simulink model "AOTRT"  (R2017b)
settings: Solver=FixedStepDiscrete  StartTime=0  StopTime=5  FixedStep=0.001  MaxStep=0.001  RelTol=1e-3  EnableMultiTasking=on
model workspace (MAT data in the model file):
  Occurrence.FaultRemote = 1
  Occurrence.FaultLow = 2
  Occurrence.FaultLow_2 = 3
  Occurrence.FaultModerate = 4
  Occurrence.FaultModerate_2 = 5
  Occurrence.FaultModerate_3 = 6
  Occurrence.FaultHigh = 7
  Occurrence.FaultHigh_2 = 8
  Occurrence.Tolerance = 9
  Occurrence.OK = 10
  Partitions.Last = ''
  Partitions.All = '*'
  Severity.OK = 0
  Severity.Warn = 1
  Severity.VeryMinor = 2
  Severity.Minor = 3
  Severity.VeryLow = 4
  Severity.Low = 5
  Severity.Moderate = 6
  Severity.High = 7
  Severity.VeryHigh = 8
  Severity.HazardousWithWarning = 9
  Severity.HazardousNoWarning = 10
  Severity.Error = 11
  Severity.ErrorFatal = 20
  block : handle (value not decoded)
  t = 0
  time = 0
libraries: EPS_lib x1
settings Model: RequirementInfo={'linktype_rmi_url' 'easee:VCC_EEDM,8630600' '' 'true' 'REQPROD 431295 / MAIN ; 5 : Actions on Torque Request timeout' '' } %GIDa_82bd7b7d_6f03_44d5_8654_a9f9591c358b  conn_id=-1  report_delay=1  Creator=aande176  LastModifiedBy=JEDDELAN
settings SolverCC: AutoInsertRateTranBlk=on
settings DataIOCC: ExternalInput=[],CPSRSts__CPSRSts,[],[],[],[],[],[],[],LvTestSts__LvTestSts,IsgPwrLimMin__IsgPwrLimMin,[],IsgPwrLimMax__IsgPwrLimMax,TqAvlIntFromIfCpt__TqAvlIntFromIfCpt,[],[],[],[],[],TqAllwdInt__TqAllwdInt,[],[],[],[],[],[],[],HvBattUDynMaxLim__HvBattUDynMaxLim,[],HvBattUDynMinLim__HvBattUDynMinLim,[],InitCmpl__InitCmpl,[],[],[],[],[],[],[],[],[],[],[],HvTestSts__HvTestSts,[],[],[],IsgModReq__IsgModReq,[],[],[],[],[],[],[],[],[],[],[],[],[],[],[],[],[],EngSt1WdSts__EngSt1WdSts__IsUpdated,IsgSpdReq__IsgSpdReq__IsUpdated,IsgModReq__IsgModReq__IsUpdated,HvSysRlySts__HvSysRlySts__IsUpdated,HvSysRlySts_toController,[],[],[],[],ImobPrpsnAllwd__ImobPrpsnAllwd__dummy,[],[],[],[],ImobTurnOffAllwd__ImobTurnOffAllwd__dummy,[],[],[],No_GearEven,B_CloseClutchOdd,B_CloseClutchEven,[],[],[],B_EnableVSpAct,V_Vehicle_SetPoint_mps,[]  SaveFormat=StructureWithTime  SaveOutput=off  SignalLogging=off  DSMLogging=off  SaveTime=off  SignalLoggingName=slunit_logdata
settings OptimizationCC: DefaultParameterBehavior=Inlined  ExpressionDepthLimit=2147483647  LifeSpan=Inf
settings DebuggingCC: RTPrefix=warning  AlgebraicLoopMsg=error  CheckSSInitialOutputMsg=off  SolverPrmCheckMsg=warning  IntegerOverflowMsg=none  ParameterPrecisionLossMsg=none  FcnCallInpInsideContextMsg=warning  BusObjectLabelMismatch=error  ModelReferenceDataLoggingMessage=none  StateNameClashWarn=warning  SFUnexpectedBacktrackingDiag=warning  SFNoUnconditionalDefaultTransitionDiag=warning  SFExecutionAtInitializationDiag=none  IntegerSaturationMsg=none
settings HardwareCC: ProdBitPerLong=64  ProdHWDeviceType=Intel->x86-64
settings ModelReferenceCC: UpdateModelReferenceTargets=AssumeUpToDate  PropagateSignalLabelsOutOfModel=off
settings SFSimCC: SimGenImportedTypeDefs=on
settings RTWCC: RTWUseSimCustomCode=on
settings CodeAppCC: StateflowObjectComments=on
settings GRTTargetCC: TargetLangStandard=C89/C90 (ANSI)  GeneratePreprocessorConditionals=Disable all  CombineOutputUpdateFcns=off  GRTInterface=on
settings ConfigComp: CovScope=Subsystem  CovPath=RequirementsEvaluation/AvailableTorque  CovMetricSettings=dcw  CovHTMLOptions=-sRT=1 -aTS=1 -bRG=1 -bTC=1 -hTR=0 -nFC=0 -scm=1 -bcm=1 -xEv=0  CovHtmlReporting=on  CovSaveCumulativeToWorkspaceVar=on  CovSaveSingleToWorkspaceVar=on  CovExternalEMLEnable=off

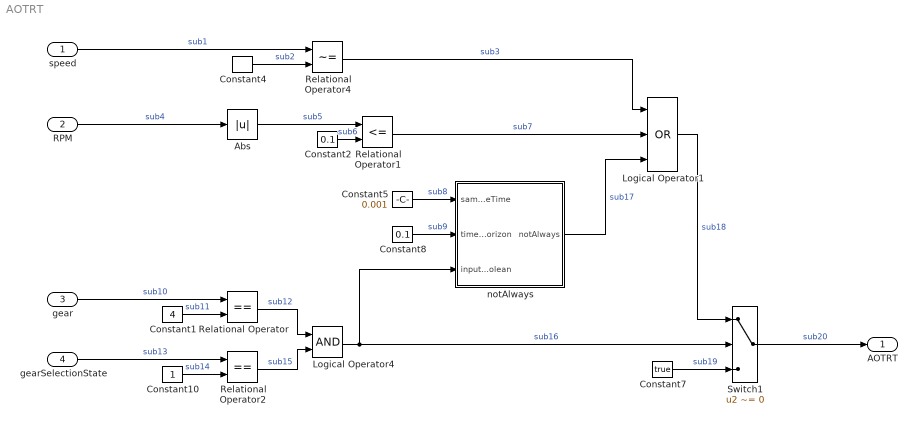
== system AOTRT ==
  speed : Inport  OutDataTypeStr=TqInt  PortDimensions=1  SampleTime=[0.001,0]
  RPM : Inport  Port=2  OutDataTypeStr=TqInt  PortDimensions=1  SampleTime=[0.001,0]
  gear : Inport  Port=3  OutDataTypeStr=Enum: ComTiOut  PortDimensions=1  SampleTime=[0.001,0]  Interpolate=off
  gearSelectionState : Inport  Port=4  OutDataTypeStr=Enum: ModSts  PortDimensions=1  SampleTime=[0.001,0]  Interpolate=off
  Abs : Abs
  Constant1 : Constant  Value=4  OutDataTypeStr=double  mask(EPS_param){param=4, displayname=4: 4}
      mask prompts: param "Parameter"; displayname "Display"
      mask help:
      | Block is used for EPS parameters.
      | Block shows the annotation 'displayname' (which is a hidden feature in the mask)
      | which is a part of the Parameter Name (if the parameter name syntax is 'ModelNameParam')
      mask init:
      | try
      |     set_param(gcb,'LinkStatus','none');
      | catch
      |     warning('Not possible to break links');
      | end
      | icondisp = 'P';
      | mdlname = regexp(get_param(gcs,'Parent'),'\w*(?=\_)','match','once');
      | name = get_param(gcb,'param');
      | 
      | objclass = evalin('base',['class(',name,')']);
      | objtype = typeobj(objclass);
      | if objtype.isenum
      |     nametype = regexp(name,'\.','split');
      | % if length(nametype) > 1
      |     % is enum
      |     displayname = nametype{2};
      |     icondisp = 'E';
      |     set_param(gcb,'OutDataTypeStr',['Enum: ',nametype{1}]);    
      | elseif isa(evalin('base',name),'AUTOSAR.Parameter')
      |     % Autosar parameter
      |     displayname = regexprep(name,mdlname,'');
      |     icondisp = 'P';
      |     set_param(gcb,'OutDataTypeStr',['Inherit: Inherit from ''Constant value''']);
      | else
      |     % regular constant
      |     displayname = [name,': ',num2str(evalin('base',name))];
      |     icondisp = 'C';
      |     if strcmp(objtype.name,'logical')
      |         set_param(gcb,'OutDataTypeStr','boolean');
      |     else
      |         set_param(gcb,'OutDataTypeStr',objtype.name);
      |     end  
      | end
      | set_param(gcb,'displayname',displayname);
      | set_param(gcb,'Value',name);
      settings: AttributesFormatString=%<displayname>
      mask Display: disp(icondisp)
  Constant10 : Constant  OutDataTypeStr=double  mask(EPS_param_v0.1){param=1, displayname=1: 1}
      mask prompts: param "Parameter"; displayname "Display"
      mask help:
      | Block is used for EPS parameters.
      | Block shows the annotation 'displayname' (which is a hidden feature in the mask)
      | which is a part of the Parameter Name (if the parameter name syntax is 'ModelNameParam')
      mask init:
      | try
      |     set_param(gcb,'LinkStatus','none');
      | catch
      |     warning('Not possible to break links');
      | end
      | icondisp = 'P';
      | mdlname = regexp(get_param(gcs,'Parent'),'\w*(?=\_)','match','once');
      | name = get_param(gcb,'param');
      | 
      | objclass = evalin('base',['class(',name,')']);
      | [enumdummy,enumList] = evalin('base',['enumeration(',name,')']);
      | if ~isempty(enumList)
      |     nametype = regexp(name,'\.','split');
      | % if length(nametype) > 1
      |     % is enum
      |     displayname = nametype{2};
      |     icondisp = 'E';
      |     set_param(gcb,'OutDataTypeStr',['Enum: ',nametype{1}]);    
      | elseif isa(evalin('base',name),'AUTOSAR.Parameter')
      |     % Autosar parameter
      |     displayname = regexprep(name,mdlname,'');
      |     icondisp = 'P';
      |     set_param(gcb,'OutDataTypeStr',['Inherit: Inherit from ''Constant value''']);
      | else
      |     % regular constant
      |     displayname = [regexprep(name,mdlname,''),': ',num2str(evalin('base',name))];
      |     icondisp = 'C';
      |     if strcmp(objclass,'logical')
      |         set_param(gcb,'OutDataTypeStr','boolean');
      |     else
      |         set_param(gcb,'OutDataTypeStr',objclass);
      |     end  
      | end
      | set_param(gcb,'displayname',displayname);
      | set_param(gcb,'Value',name);
      settings: AttributesFormatString=%<displayname>
      mask Display: disp(icondisp)
  Constant2 : Constant  Value=0.1  OutDataTypeStr=double  mask(EPS_param_v0.1){param=0.1, displayname=0.1: 0.1}
      mask prompts: param "Parameter"; displayname "Display"
      mask help:
      | Block is used for EPS parameters.
      | Block shows the annotation 'displayname' (which is a hidden feature in the mask)
      | which is a part of the Parameter Name (if the parameter name syntax is 'ModelNameParam')
      mask init: same as AOTRT/Constant10
      settings: AttributesFormatString=%<displayname>
      mask Display: disp(icondisp)
  Constant4 : EPS_lib/CalibrationAndMeasurement/Constant  param=0  displayname=0: 0
      settings: AttributesFormatString=%<displayname>  SourceProductName=EPS library
  Constant5 : Constant  Value=0.001  OutDataTypeStr=double  mask(EPS_param){param=0.001, displayname=0.001: 0.001}
      mask prompts: param "Parameter"; displayname "Display"
      mask help:
      | Block is used for EPS parameters.
      | Block shows the annotation 'displayname' (which is a hidden feature in the mask)
      | which is a part of the Parameter Name (if the parameter name syntax is 'ModelNameParam')
      mask init: same as AOTRT/Constant1
      settings: AttributesFormatString=%<displayname>
      mask Display: disp(icondisp)
  Constant7 : Constant  Value=true  OutDataTypeStr=boolean  mask(EPS_param){param=true, displayname=true: 1}
      mask prompts: param "Parameter"; displayname "Display"
      mask help:
      | Block is used for EPS parameters.
      | Block shows the annotation 'displayname' (which is a hidden feature in the mask)
      | which is a part of the Parameter Name (if the parameter name syntax is 'ModelNameParam')
      mask init: same as AOTRT/Constant1
      settings: AttributesFormatString=%<displayname>
      mask Display: disp(icondisp)
  Constant8 : Constant  Value=0.1  OutDataTypeStr=double  mask(EPS_param){param=0.1, displayname=0.1: 0.1}
      mask prompts: param "Parameter"; displayname "Display"
      mask help:
      | Block is used for EPS parameters.
      | Block shows the annotation 'displayname' (which is a hidden feature in the mask)
      | which is a part of the Parameter Name (if the parameter name syntax is 'ModelNameParam')
      mask init: same as AOTRT/Constant1
      settings: AttributesFormatString=%<displayname>
      mask Display: disp(icondisp)
  Logical Operator1 : Logic  Operator=OR  Inputs=3  AllPortsSameDT=off  OutDataTypeStr=boolean
  Logical Operator4 : Logic  AllPortsSameDT=off  OutDataTypeStr=boolean
  Relational Operator : RelationalOperator  Operator===  OutDataTypeStr=boolean  RndMeth=Nearest
  Relational Operator1 : RelationalOperator  Operator=<=  OutDataTypeStr=boolean  RndMeth=Nearest
  Relational Operator2 : RelationalOperator  Operator===  OutDataTypeStr=boolean  RndMeth=Nearest
  Relational Operator4 : RelationalOperator  Operator=~=  OutDataTypeStr=boolean  RndMeth=Nearest
  Switch1 : Switch  Criteria=u2 ~= 0
  notAlways : Subsystem
      settings: CopyFcn=set_param(gcbh,'LinkStatus','none');
  AOTRT : Outport  OutDataTypeStr=boolean  PortDimensions=1  SampleTime=[0.001,0]
  wires:
  Relational Operator4/1 -> Logical Operator1/1  "sub3"
  Constant4/1 -> Relational Operator4/2  "sub2"
  speed/1 -> Relational Operator4/1  "sub1"
  Constant2/1 -> Relational Operator1/2  "sub6"
  Relational Operator2/1 -> Logical Operator4/2  "sub15"
  Constant10/1 -> Relational Operator2/2  "sub14"
  gearSelectionState/1 -> Relational Operator2/1  "sub13"
  Logical Operator4/1 -> notAlways/3(inputBoolean), Switch1/2  "sub16"
  Relational Operator/1 -> Logical Operator4/1  "sub12"
  Constant5/1 -> notAlways/1(sampleTime)  "sub8"
  Constant8/1 -> notAlways/2(timeHorizon)  "sub9"
  notAlways/1(notAlways) -> Logical Operator1/3  "sub17"
  Constant7/1 -> Switch1/3  "sub19"
  Logical Operator1/1 -> Switch1/1  "sub18"
  Relational Operator1/1 -> Logical Operator1/2  "sub7"
  Abs/1 -> Relational Operator1/1  "sub5"
  RPM/1 -> Abs/1  "sub4"
  Constant1/1 -> Relational Operator/2  "sub11"
  gear/1 -> Relational Operator/1  "sub10"
  Switch1/1 -> AOTRT/1  "sub20"

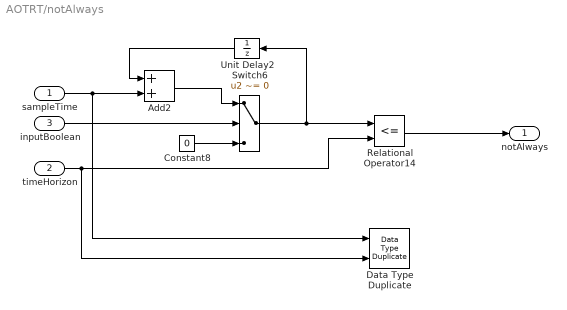
== system AOTRT/notAlways ==
  sampleTime : Inport
  timeHorizon : Inport  Port=2
  inputBoolean : Inport  Port=3
  Add2 : Sum
  Constant8 : Constant  Value=0  OutDataTypeStr=Inherit: Inherit via back propagation
  Data Type Duplicate : DataTypeDuplicate
  Relational Operator14 : RelationalOperator  Operator=<=  OutDataTypeStr=boolean  RndMeth=Nearest
  Switch6 : Switch  Criteria=u2 ~= 0
  Unit Delay2 : UnitDelay  SampleTime=-1
  notAlways : Outport
  wires:
  Switch6/1 -> Relational Operator14/1, Unit Delay2/1
  timeHorizon/1 -> Relational Operator14/2, Data Type Duplicate/2
  Relational Operator14/1 -> notAlways/1
  Unit Delay2/1 -> Add2/1
  Add2/1 -> Switch6/1
  sampleTime/1 -> Add2/2, Data Type Duplicate/1
  Constant8/1 -> Switch6/3
  inputBoolean/1 -> Switch6/2
